simulink model "sampleModel1454"  (R2023a)
settings: Solver=VariableStepAuto  StartTime=0.0  StopTime=10.0  RelTol=1e-3
libraries: hdlsllib x7, simulink x1
settings Model: Creator=user1  LastModifiedBy=user1

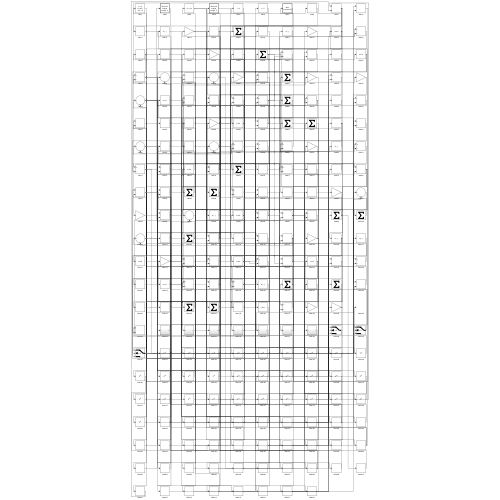
[thumbnail: Simulink's stored preview of the top-level diagram]
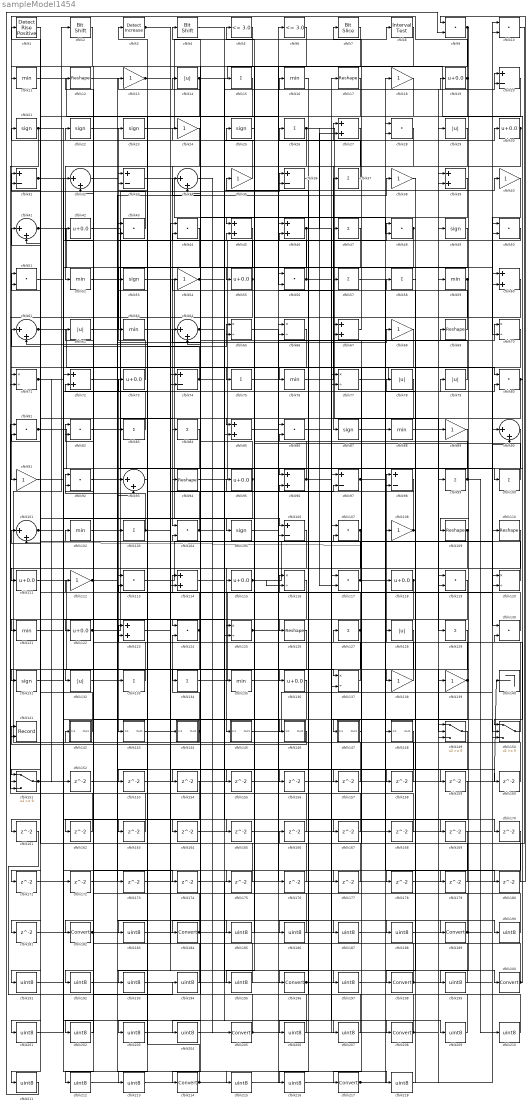
== system sampleModel1454 ==
  cfblk1 : hdlsllib/Logic and Bit Operations/Detect Rise Positive  vinit=0  OutDataTypeStr=boolean
  cfblk{9..10,28,43..44,48,50..51,56,80..82,86,92,104,107,113,117,119,124,130} (21 alike) : DotProduct  OutDataTypeStr=Inherit: Inherit via internal rule
  cfblk{15,26,37,47,57..58,75,83..84,99..100,103,127,129,133..134} (16 alike) : Sum  Inputs=+
  cfblk{32,34,41,61,64,90,93,101} (8 alike) : Sum  Inputs=|++
  cfblk{11,16,52,59,63,76,88,102,121,135} (10 alike) : MinMax
  cfblk{21..23,25,49,53,87,105,131} (9 alike) : Signum
  cfblk{20,31,33,36,74,97..98,106} (8 alike) : Sum  Inputs=+-
  cfblk{13,18,24,35,38,40,54,68,89,91,108,112,138..139} (14 alike) : Gain
  cfblk{12,17,69,94,109..110,126} (7 alike) : Reshape
  cfblk{19,30,42,55,73,95,111,115,118,122,136} (11 alike) : Bias  Bias=0.0  SaturateOnIntegerOverflow=off
  cfblk{27,39,45..46,60,67,72,85,96,114,123} (11 alike) : Sum
  cfblk{65..66,70..71,77,116,120,125,137} (9 alike) : Product  Inputs=*/  RndMeth=Zero  SaturateOnIntegerOverflow=on
  cfblk{14,29,62,78..79,128,132} (7 alike) : Abs  SaturateOnIntegerOverflow=off
  cfblk140 : Terminator
  cfblk141 : Record  FileSettingsInternal="{\"entries\":[{\"content\":{\"excelSettings\":{\"content\":{},\"type\":\"Streamout.ExcelSettings\"}},\"type\":\"Streamout.FileSettingStorage\",\"uuid\":\"\"}],\"packageUris\":[\"http:\\/\\/schema.mathworks.com\\/mf0\\/streamout_blocks\\/R2020a\"],\"version\":\"1.0\"}"  Layout=[1 1]  SignalsInternal="{\"entries\":[{\"content\":{\"signals\":[{\"content\":{\"blockPath\":[],\"dimensions\":[1],\"domain\":\"\",\"lineColor\":\"#a2142f\",\"plots\":[1],\"port\":1,\"signalID\":780,\"signalName\":\"XY Graph:1\"},\"type\":\"RecordBlkView.Signal\",\"uuid\":\"\"},{\"content\":{\"blockPath\":[],\"dimensions\":[1],\"domain\":\"\",\"lineColor\":\"#139fff\",\"plots\":[1],\"port\":2,\"signalID\":783,\"signalName\":\"XY Graph:2\"},\"type\":\"RecordBlkView.Signal\",\"uuid\":\"\"}]},\"type\":\"RecordBlkView.InputSignals\",\"uuid\":\"\"}],\"packageUris\":[\"http:\\/\\/schema.mathworks.com\\/mf0\\/streamout_blocks\\/R2020a\"],\"version\":\"1.0\"}"  VisualizationBindings="{\"xyplotplugin\":{\"info\":[{\"series\":[{\"bindingParametersList\":[{\"parameter\":\"X-Axis\",\"signalID\":780,\"signalName\":\"XY Graph:1\"},{\"parameter\":\"Y-Axis\",\"signalID\":783,\"signalName\":\"XY Graph:2\"}],\"seriesID\":49486}],\"subplotID\":1}]}}"  CompatibilityTag=XY  st=-1
  cfblk142 : Subsystem
      settings: LibrarySourceBlock=|
      | hdlsllib/Ports &
      | Subsystems/Subsystem
  cfblk143 : Subsystem
      settings: LibrarySourceBlock=|
      | hdlsllib/Ports &
      | Subsystems/Subsystem
  cfblk144 : Subsystem
      settings: LibrarySourceBlock=|
      | hdlsllib/Ports &
      | Subsystems/Subsystem
  cfblk145 : Subsystem
      settings: LibrarySourceBlock=|
      | hdlsllib/Ports &
      | Subsystems/Subsystem
  cfblk146 : Subsystem
      settings: LibrarySourceBlock=|
      | hdlsllib/Ports &
      | Subsystems/Subsystem
  cfblk147 : Subsystem
      settings: LibrarySourceBlock=|
      | hdlsllib/Ports &
      | Subsystems/Subsystem
  cfblk148 : Subsystem
      settings: LibrarySourceBlock=|
      | hdlsllib/Ports &
      | Subsystems/Subsystem
  cfblk149 : Switch  SaturateOnIntegerOverflow=off  InputSameDT=off
  cfblk150 : Switch  SaturateOnIntegerOverflow=off  InputSameDT=off
  cfblk151 : Switch  SaturateOnIntegerOverflow=off  InputSameDT=off
  cfblk{152..181} (30 alike) : Delay  SampleTime=1
  cfblk{182,184,189,196,198,200,205,208,214,217} (10 alike) : DataTypeConversion  SaturateOnIntegerOverflow=off  RndMeth=Floor
  cfblk{183,185..188,190..195,197,199,201..204,206..207,209..213,215..216,218} (27 alike) : DataTypeConversion  OutDataTypeStr=uint8  SaturateOnIntegerOverflow=off  RndMeth=Floor
  cfblk2 : hdlsllib/Logic and Bit Operations/Bit Shift  mode=Shift Left Logical  N=0
  cfblk3 : simulink/Logic and Bit Operations/Detect Increase  vinit=0.0  OutDataTypeStr=boolean
      settings: LibrarySourceBlock=|
      | hdlsllib/Logic and Bit
      | Operations/Detect
      | Increase
  cfblk4 : hdlsllib/Logic and Bit Operations/Bit Shift  mode=Shift Left Logical  N=0
  cfblk5 : hdlsllib/Logic and Bit Operations/Compare To Constant  relop=<=  const=3.0  OutDataTypeStr=boolean
  cfblk6 : hdlsllib/Logic and Bit Operations/Compare To Constant  relop=<=  const=3.0  OutDataTypeStr=boolean
  cfblk7 : hdlsllib/Logic and Bit Operations/Bit Slice  lidx=7  ridx=0
  cfblk8 : hdlsllib/Logic and Bit Operations/Interval Test  IntervalClosedRight=on  uplimit=0.5  IntervalClosedLeft=on  lowlimit=-0.5  OutDataTypeStr=boolean
  wires:
  cfblk63/1 -> cfblk105/1
  cfblk24/1 -> cfblk52/1
  cfblk73/1 -> cfblk23/1
  cfblk101/1 -> cfblk134/1, cfblk174/1
  cfblk23/1 -> cfblk8/1
  cfblk99/1 -> cfblk35/1, cfblk210/1
  cfblk80/1 -> cfblk132/1, cfblk150/1, cfblk177/1
  cfblk77/1 -> cfblk80/1
  cfblk19/1 -> cfblk91/1, cfblk45/1, cfblk85/2
  cfblk30/1 -> cfblk87/1, cfblk124/1
  cfblk144/1(Out1) -> cfblk2/1, cfblk124/2
  cfblk3/1 -> cfblk188/1, cfblk190/1
  cfblk36/1 -> cfblk96/1
  cfblk85/1 -> cfblk70/1
  cfblk103/1 -> cfblk92/1, cfblk97/2
  cfblk121/1 -> cfblk72/1
  cfblk68/1 -> cfblk147/1(In1)
  cfblk14/1 -> cfblk100/1, cfblk83/1
  cfblk2/1 -> cfblk11/1
  cfblk150/1 -> cfblk98/1
  cfblk26/1 -> cfblk129/1, cfblk117/2, cfblk114/2
  cfblk28/1 -> cfblk104/1
  cfblk84/1 -> cfblk143/1(In1)
  cfblk128/1 -> cfblk217/1
  cfblk81/1 -> cfblk120/1, cfblk65/2
  cfblk71/1 -> cfblk106/2, cfblk152/1
  cfblk122/1 -> cfblk36/1, cfblk116/1
  cfblk107/1 -> cfblk101/2, cfblk201/1
  cfblk76/1 -> cfblk37/1
  cfblk94/1 -> cfblk48/1
  cfblk100/1 -> cfblk25/1
  cfblk40/1 -> cfblk70/2
  cfblk70/1 -> cfblk111/1
  cfblk109/1 -> cfblk145/1(In1), cfblk125/1
  cfblk25/1 -> cfblk115/1
  cfblk127/1 -> cfblk101/1, cfblk42/1, cfblk131/1
  cfblk55/1 -> cfblk43/1, cfblk71/2
  cfblk43/1 -> cfblk31/1
  cfblk72/1 -> cfblk93/1
  cfblk58/1 -> cfblk198/1
  cfblk124/1 -> cfblk114/1, cfblk161/1
  cfblk67/1 -> cfblk7/1
  cfblk56/1 -> cfblk4/1, cfblk19/1
  cfblk83/1 -> cfblk22/1
  cfblk133/1 -> cfblk123/1
  cfblk134/1 -> cfblk10/1
  cfblk129/1 -> cfblk149/2
  cfblk102/1 -> cfblk189/1
  cfblk86/1 -> cfblk208/1
  cfblk97/1 -> cfblk80/2, cfblk179/1
  cfblk53/1 -> cfblk97/1
  cfblk29/1 -> cfblk55/1
  cfblk111/1 -> cfblk137/1
  cfblk118/1 -> cfblk123/2, cfblk151/3
  cfblk61/1 -> cfblk130/1, cfblk146/1(In1)
  cfblk79/1 -> cfblk13/1
  cfblk87/1 -> cfblk108/1
  cfblk1/1 -> cfblk121/1
  cfblk33/1 -> cfblk48/2
  cfblk46/1 -> cfblk27/2, cfblk150/2, cfblk195/1
  cfblk42/1 -> cfblk94/1
  cfblk32/1 -> cfblk200/1
  cfblk148/1(Out1) -> cfblk196/1
  cfblk113/1 -> cfblk17/1
  cfblk64/1 -> cfblk30/1, cfblk170/1
  cfblk9/1 -> cfblk56/2, cfblk64/2, cfblk199/1
  cfblk108/1 -> cfblk24/1, cfblk138/1
  cfblk31/1 -> cfblk125/2, cfblk165/1
  cfblk52/1 -> cfblk84/1
  cfblk54/1 -> cfblk76/1, cfblk40/1
  cfblk20/1 -> cfblk122/1
  cfblk139/1 -> cfblk78/1, cfblk192/1
  cfblk18/1 -> cfblk74/2
  cfblk74/1 -> cfblk71/1, cfblk16/1, cfblk33/2
  cfblk59/1 -> cfblk109/1, cfblk75/1
  cfblk130/1 -> cfblk51/1
  cfblk146/1(Out1) -> cfblk141/1
  cfblk13/1 -> cfblk106/1, cfblk77/2
  cfblk21/1 -> cfblk151/2, cfblk169/1
  cfblk114/1 -> cfblk27/1
  cfblk49/1 -> cfblk126/1
  cfblk37/1 -> cfblk26/1
  cfblk115/1 -> cfblk60/1, cfblk116/2
  cfblk147/1(Out1) -> cfblk127/1
  cfblk16/1 -> cfblk136/1
  cfblk7/1 -> cfblk135/1
  cfblk112/1 -> cfblk68/1, cfblk38/1
  cfblk151/1 -> cfblk10/2, cfblk140/1, cfblk90/2, cfblk167/1
  cfblk34/1 -> cfblk205/1
  cfblk6/1 -> cfblk182/1
  cfblk39/1 -> cfblk214/1
  cfblk62/1 -> cfblk144/1(In1)
  cfblk48/1 -> cfblk43/2, cfblk164/1
  cfblk142/1(Out1) -> cfblk81/2
  cfblk104/1 -> cfblk61/2, cfblk20/2, cfblk53/1
  cfblk35/1 -> cfblk21/1
  cfblk145/1(Out1) -> cfblk110/1
  cfblk116/1 -> cfblk133/1
  cfblk4/1 -> cfblk47/1
  cfblk5/1 -> cfblk184/1
  cfblk125/1 -> cfblk118/1, cfblk57/1
  cfblk110/1 -> cfblk141/2
  cfblk135/1 -> cfblk69/1
  cfblk98/1 -> cfblk96/2
  cfblk120/1 -> cfblk67/1
  cfblk11/1 -> cfblk56/1
  cfblk69/1 -> cfblk54/1
  cfblk117/1 -> cfblk41/2, cfblk180/1
  cfblk95/1 -> cfblk64/1, cfblk151/1
  cfblk138/1 -> cfblk33/1
  cfblk50/1 -> cfblk46/2
  cfblk45/1 -> cfblk63/1
  cfblk96/1 -> cfblk65/1, cfblk158/1
  cfblk131/1 -> cfblk79/1
  cfblk41/1 -> cfblk103/1, cfblk45/2, cfblk60/2, cfblk98/2
  cfblk17/1 -> cfblk85/1
  cfblk137/1 -> cfblk82/1
  cfblk88/1 -> cfblk20/1
  cfblk152/1 -> cfblk50/2
  cfblk106/1 -> cfblk153/1
  cfblk153/1 -> cfblk74/1
  cfblk47/1 -> cfblk154/1
  cfblk60/1 -> cfblk155/1
  cfblk155/1 -> cfblk46/1
  cfblk123/1 -> cfblk156/1
  cfblk156/1 -> cfblk137/2
  cfblk22/1 -> cfblk157/1
  cfblk157/1 -> cfblk113/1
  cfblk158/1 -> cfblk104/2
  cfblk65/1 -> cfblk159/1
  cfblk105/1 -> cfblk160/1
  cfblk160/1 -> cfblk28/1
  cfblk27/1 -> cfblk162/1
  cfblk162/1 -> cfblk61/1
  cfblk90/1 -> cfblk163/1
  cfblk163/1 -> cfblk41/1
  cfblk164/1 -> cfblk149/3
  cfblk165/1 -> cfblk120/2
  cfblk10/1 -> cfblk166/1
  cfblk166/1 -> cfblk92/2
  cfblk167/1 -> cfblk31/2
  cfblk57/1 -> cfblk168/1
  cfblk168/1 -> cfblk81/1
  cfblk78/1 -> cfblk171/1
  cfblk171/1 -> cfblk93/2
  cfblk172/1 -> cfblk72/2
  cfblk12/1 -> cfblk173/1
  cfblk173/1 -> cfblk9/1
  cfblk8/1 -> cfblk175/1
  cfblk175/1 -> cfblk1/1
  cfblk75/1 -> cfblk176/1
  cfblk176/1 -> cfblk51/2
  cfblk177/1 -> cfblk77/1
  cfblk38/1 -> cfblk178/1
  cfblk178/1 -> cfblk149/1
  cfblk179/1 -> cfblk67/2
  cfblk180/1 -> cfblk107/2
  cfblk126/1 -> cfblk181/1
  cfblk181/1 -> cfblk49/1
  cfblk182/1 -> cfblk90/1, cfblk62/1
  cfblk136/1 -> cfblk183/1
  cfblk183/1 -> cfblk6/1
  cfblk184/1 -> cfblk59/1, cfblk73/1
  cfblk132/1 -> cfblk185/1
  cfblk185/1 -> cfblk5/1
  cfblk119/1 -> cfblk186/1
  cfblk186/1 -> cfblk14/1
  cfblk82/1 -> cfblk187/1
  cfblk187/1 -> cfblk119/1
  cfblk188/1 -> cfblk119/2
  cfblk189/1 -> cfblk12/1, cfblk95/1
  cfblk190/1 -> cfblk102/1
  cfblk15/1 -> cfblk191/1
  cfblk191/1 -> cfblk172/1
  cfblk192/1 -> cfblk15/1
  cfblk44/1 -> cfblk193/1
  cfblk193/1 -> cfblk18/1
  cfblk161/1 -> cfblk194/1
  cfblk194/1 -> cfblk44/1
  cfblk195/1 -> cfblk44/2
  cfblk196/1 -> cfblk150/3, cfblk139/1
  cfblk143/1(Out1) -> cfblk197/1
  cfblk197/1 -> cfblk148/1(In1)
  cfblk198/1 -> cfblk29/1, cfblk107/1
  cfblk199/1 -> cfblk58/1
  cfblk200/1 -> cfblk130/2, cfblk36/2, cfblk142/1(In1)
  cfblk201/1 -> cfblk32/1
  cfblk154/1 -> cfblk202/1
  cfblk202/1 -> cfblk32/2
  cfblk89/1 -> cfblk203/1
  cfblk203/1 -> cfblk28/2
  cfblk149/1 -> cfblk204/1
  cfblk204/1 -> cfblk89/1
  cfblk205/1 -> cfblk82/2, cfblk117/1
  cfblk170/1 -> cfblk206/1
  cfblk206/1 -> cfblk34/1
  cfblk51/1 -> cfblk207/1
  cfblk207/1 -> cfblk34/2
  cfblk208/1 -> cfblk112/1, cfblk3/1
  cfblk174/1 -> cfblk209/1
  cfblk209/1 -> cfblk86/1
  cfblk210/1 -> cfblk86/2
  cfblk66/1 -> cfblk211/1
  cfblk211/1 -> cfblk9/2
  cfblk169/1 -> cfblk212/1
  cfblk212/1 -> cfblk66/1
  cfblk93/1 -> cfblk213/1
  cfblk213/1 -> cfblk66/2
  cfblk214/1 -> cfblk88/1, cfblk113/2
  cfblk91/1 -> cfblk215/1
  cfblk215/1 -> cfblk39/1
  cfblk159/1 -> cfblk216/1
  cfblk216/1 -> cfblk39/2
  cfblk217/1 -> cfblk99/1, cfblk50/1
  cfblk92/1 -> cfblk218/1
  cfblk218/1 -> cfblk128/1

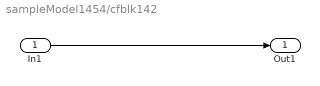
== system sampleModel1454/cfblk142 ==
  In1 : Inport
  Out1 : Outport
  wires:
  In1/1 -> Out1/1

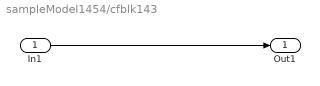
== system sampleModel1454/cfblk143 ==
  In1 : Inport
  Out1 : Outport
  wires:
  In1/1 -> Out1/1

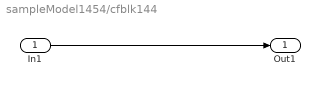
== system sampleModel1454/cfblk144 ==
  In1 : Inport
  Out1 : Outport
  wires:
  In1/1 -> Out1/1

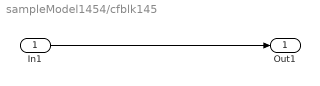
== system sampleModel1454/cfblk145 ==
  In1 : Inport
  Out1 : Outport
  wires:
  In1/1 -> Out1/1

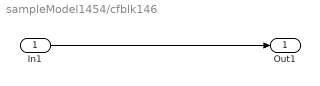
== system sampleModel1454/cfblk146 ==
  In1 : Inport
  Out1 : Outport
  wires:
  In1/1 -> Out1/1

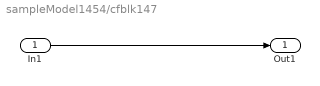
== system sampleModel1454/cfblk147 ==
  In1 : Inport
  Out1 : Outport
  wires:
  In1/1 -> Out1/1

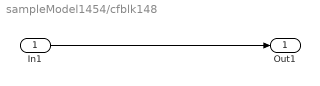
== system sampleModel1454/cfblk148 ==
  In1 : Inport
  Out1 : Outport
  wires:
  In1/1 -> Out1/1
